simulink model "LabFabSim2022a__2_9_2023_AllAttacks_"  (R2022a)
settings: Solver=VariableStepAuto  StartTime=0.0  StopTime=5500000  RelTol=1e-3  EnableMultiTasking=on
model workspace (MAT data in the model file):
  JsonData : timetable (value not decoded)
  M : Simulink.Parameter (value not decoded)
  ROS_trigger = 0
  SL_ROS_VariableLengthArrays_MaxSizes : object (value not decoded)
undefined symbols (not defined in the file): DOS, DOSinitGen, DTP, DTPGen, DTPInitGen, EmptyLocFound, InitCobot, InitCobotReturn, InitializeSLD, InitLEGO, InitVGRproc2, m, MC, MCGen, MCInitGen, MO, MOGen, MOInitGen, n, NetScan, NetScanInitGen, Spying, SpyingInitGen, WS, WSGen, WSInitGen
libraries: sldelib x6
(part 3 of 4)

== system LabFabSim2022a__2_9_2023_AllAttacks_/VGR_Proc3 (Ramp) ==
  note: Published Return Postion
  note: DPS Detected <color> object
  note: VGR is Moving to DPS Color Sensor
  note: VGR is Picking Up Material from in-Processing Unit
  note: Calling cobot for <color> pick up
  LEGO_Cobot : Inport
  Cobot moves to pickup parts at the end of LEGO Process : EntityServer  InputPortMessageModes=m  OutputPortMessageModes=m  Capacity=1  ServiceTimeSource=Attribute  ServiceTimeAttributeName=LEGO_ServiceTime  EntryAction=|
      | sourceID(5); %lego
      | sourceAddress(4); %/lego_node
      | sourceType(1); %motion sensor
      | sourceLocation(2); %Expansion
      | destinationServiceAddress(5); %/listener(cobot)
      | destinationServiceType(5); %next task
      | destinationServiceLocation(2); %Expansion
      | accessedNodeAddress(4); 
      | accessedNodeType(1); %String
      | operation(3); %notify-callback
      | Normality(1); %normal
      | 
      | if entity.ColorID == 1
      |     value(38); %Calling cobot for RED pick up
      | else if entity.ColorID == 2
      |     value(39); %Calling cobot for BLUE pick up
      | else 
      |     value(40); %Calling cobot for WHITE pick up
      | end
  ColorSensor2 requests an open pos in HBW : EntityServer  InputPortMessageModes=m  OutputPortMessageModes=m  Capacity=1  ServiceTimeValue=5  ServiceCompleteAction=|
      | sourceID(2); %vgr
      | sourceAddress(2); %/vgr_node
      | sourceType(2); %Color sensor 
      | sourceLocation(1); %Fischertechnik
      | destinationServiceAddress(3); %/status update (main)
      | destinationServiceType(5); %next task
      | destinationServiceLocation(1); %Fischertechnik
      | accessedNodeAddress(3); 
      | accessedNodeType(1); %string
      | operation(3); %notify-callback
      | Normality(1); %normal
      | 
      | if entity.ColorID == 1
      |     value(25); %DPS Detectied RED object 
      | else if entity.ColorID == 2
      |     value(24); %DPS Detected BLUE Object 
      | else
      |     value(26); %DPS Detected WHITE object
      | end
  Empty Loc returned : EntityServer  InputPortMessageModes=m  OutputPortMessageModes=m  Capacity=1  ServiceTimeValue=0.2  EntryAction=EmptyLocFound();  ServiceCompleteAction=|
      | sourceID(3); %main
      | sourceAddress(3); %/status_update (main)
      | sourceType(4); %Order
      | sourceLocation(1); %FischerTechnik
      | destinationServiceAddress(2); %vgr_node
      | destinationServiceType(5); %Next Task
      | destinationServiceLocation(1); %Fischertechnik
      | accessedNodeAddress(2);
      | accessedNodeType(1); %string
      | operation(1); %read
      | value(43); %Published Return Postion
      | Normality(1); %normal
  Entity Gate : EntityGate  InputPortMessageModes=m,m  OutputPortMessageModes=m  OperatingMode=Release gate
  "Pump off; Cobot returns home and VGR picks up part " : EntityServer  InputPortMessageModes=m  OutputPortMessageModes=m  Capacity=1  ServiceTimeValue=3  ExitAction=|
      | sourceID(2); %vgr
      | sourceAddress(2); %/vgr_node
      | sourceType(1); %motion sensor
      | sourceLocation(1); %Fischertechnik
      | destinationServiceAddress(2); %/vgr_node
      | destinationServiceType(5); %next task
      | destinationServiceLocation(1); %Fischertechnik
      | accessedNodeAddress(3); 
      | accessedNodeType(2); %Boolean
      | operation(3); %notify-callback
      | value(22); %VGR is Picking Up Material from in-Processing Unit
      | Normality(1); %normal
  Pump on; Moves to VGR Ramp : EntityServer  InputPortMessageModes=m  OutputPortMessageModes=m  Capacity=1  ServiceTimeValue=10
  Simulink Function : Subsystem  TreatAsAtomicUnit=on
  VGR moves to color sensor 2 : EntityServer  InputPortMessageModes=m  OutputPortMessageModes=m  Capacity=1  ServiceTimeValue=11  ExitAction=|
      | sourceID(2); %vgr
      | sourceAddress(2); %/vgr_node
      | sourceType(5); %next task
      | sourceLocation(1); %Fischertechnik
      | destinationServiceAddress(2); %/vgr_node
      | destinationServiceType(5); %next task
      | destinationServiceLocation(1); %Fischertechnik
      | accessedNodeAddress(3); 
      | accessedNodeType(1); %string
      | operation(3); %notify-callback
      | value(23); %VGR is Moving to DPS Color Sensor
      | Normality(1); %normal
  Cobot_VGR : Outport
  wires:
  Cobot moves to pickup parts at the end of LEGO Process/1 -> Pump on; Moves to VGR Ramp/1
  LEGO_Cobot/1 -> Cobot moves to pickup parts at the end of LEGO Process/1
  Pump on; Moves to VGR Ramp/1 -> "Pump off; Cobot returns home and VGR picks up part "/1
  "Pump off; Cobot returns home and VGR picks up part "/1 -> VGR moves to color sensor 2/1
  ColorSensor2 requests an open pos in HBW/1 -> Empty Loc returned/1
  Empty Loc returned/1 -> Entity Gate/2
  Simulink Function/1(Out1) -> Entity Gate/1
  Entity Gate/1 -> Cobot_VGR/1
  VGR moves to color sensor 2/1 -> ColorSensor2 requests an open pos in HBW/1

== system LabFabSim2022a__2_9_2023_AllAttacks_/WrongSetup (WS) ==
  note: SourID(2), SourAdd(2), SourType(3), SourLoc(1), Dest.Serv.Add(4), Dest.Serv.Type(1), Dest.Serv.Loc(2), Acc.Node.Add(4), Acc.Node.Type(2), Op(1), Val(48)
  note: Entity Gate:
      | set to open when a positive signal value is passed into the control port. Closes when negative.
  note: Recieve signal from Chance-setting Server block for activation signal
  note: Service Time: 1700 Timestep
  note: Generates a single entity that causes Wrong Setup attack (entity generator) to generate one entity
  note: Sets WS_id up to 6 and resets to 1 for next Wrong Setup attack
  note: On Service Completion: Send a signal to data-logging SimFunctions
  note: Service Time: 600 Timestep
  Display : Display
  Entity Gate : EntityGate  InputPortMessageModes=m,m  OutputPortMessageModes=m
  Entity Generator : EntityGenerator  InputPortMessageModes=m  OutputPortMessageModes=m  GenerationMethod=Event-based  IntergenerationTimeAction=|  GenerateAction=|  AttributeName=WS_id  EntityType=Structured  EntityTypeName=WSAttack
      IntergenerationTimeAction=|
      | chanceDOS = rand(1,1);
      | if chanceDOS < 0.3
      |     dt = 1
      GenerateAction=|
      | persistent next_id_WS
      | 
      | if isempty(next_id_WS)
      |     next_id_WS = 1;
      |     %set seed for random number generation
      |     rng(12345);
      | end
      | 
      | entity.WS_id = next_id_WS
      | next_id_WS = next_id_WS + 1
      | 
      | if entity.WS_id == 1
      |     next_id_WS = 1
      settings: InputPortMap=u0
  Entity Server : EntityServer  InputPortMessageModes=m  OutputPortMessageModes=m  Capacity=1  ServiceTimeValue=1700  ServiceCompleteAction=|
      | sourceID(2); %vgr
      | sourceAddress(2); %/vgr_node
      | sourceType(3); %Reference Switch
      | sourceLocation(1); %Fischertechnik
      | destinationServiceAddress(4); %/lego_node
      | destinationServiceType(1); %Motion Sensor
      | destinationServiceLocation(2); %Expansion
      | accessedNodeAddress(4); 
      | accessedNodeType(2); %Boolean
      | operation(1); %read
      | value(44); %False
      | Normality(3); %anomalous(wrongSetUp)
  Entity Server1 : EntityServer  InputPortMessageModes=m  OutputPortMessageModes=m  Capacity=1  ServiceTimeValue=600  ServiceCompleteAction=|
      | sourceID(2); %vgr
      | sourceAddress(2); %/vgr_node
      | sourceType(3); %Reference Switch
      | sourceLocation(1); %Fischertechnik
      | destinationServiceAddress(4); %/lego_node
      | destinationServiceType(1); %Motion Sensor
      | destinationServiceLocation(2); %Expansion
      | accessedNodeAddress(4); 
      | accessedNodeType(2); %Boolean
      | operation(1); %read
      | value(44); %Flase
      | Normality(3); %anomalous(wrongSetUp)
  Entity Store : EntityStore  InputPortMessageModes=m  OutputPortMessageModes=m  Capacity=2
      settings: OutputPortMap=o4
  Entity Terminator1 : EntityTerminator  InputPortMessageModes=m  NumberEntitiesArrived=on
      settings: OutputPortMap=o0
  InitWrongSetup : Subsystem
  "Number of Entities Generated from main " : Display
  Simulink Function1 : Subsystem  TreatAsAtomicUnit=on
  Subsystem1 : Subsystem
  Wrong Setup : Subsystem  TreatAsAtomicUnit=on
  wires:
  Simulink Function1/1(Out1) -> Entity Generator/1
  Entity Terminator1/1 -> Display/1
  Entity Generator/1 -> Entity Store/1
  Entity Store/1 -> Entity Gate/2
  Entity Server/1 -> Entity Server1/1
  Wrong Setup/1(Out1) -> Entity Gate/1
  Subsystem1/1(Out1) -> Simulink Function1/1(In1)
  InitWrongSetup/1(Out1) -> "Number of Entities Generated from main "/1
  Entity Server1/1 -> Entity Terminator1/1
  Entity Gate/1 -> Entity Server/1

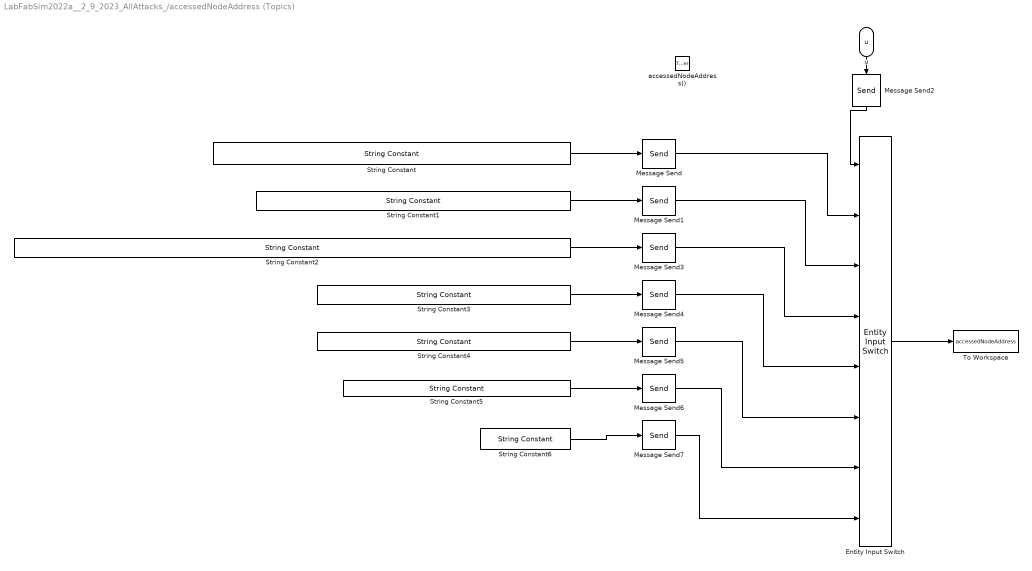
== system LabFabSim2022a__2_9_2023_AllAttacks_/accessedNodeAddress (Topics) ==
  accessedNodeAddress() : TriggerPort  TriggerType=function-call  IsSimulinkFunction=on  FunctionName=accessedNodeAddress  VariantControl=(inherit)
  Entity Input Switch : EntityInputSwitch  InputPortMessageModes=m,m,m,m,m,m,m,m  OutputPortMessageModes=m  NumberInputPorts=7  ActivePortSelection=Switch  SwitchingCriterion=From control port
      settings: InputPortMap=u0,u1,u2,u3,u4,u5,u6,u7
  Message Send{,1..7} (8 alike) : Send  OutputPortMessageModes=m
  String Constant : StringConstant  String="\"/diagnostics, /hbw_pub, /new_order, /rosout, /vgr_new_material, /what_is_empty, /what_is_occupied\""
  String Constant1 : StringConstant  String="\"/provide_empty_loc, /provide_empty_loc_back, /rosout, /what_is_empty, /what_is_occupied\""
  String Constant2 : StringConstant  String="\"/diagnostics, /new_order, /provide_empty_loc, /provide_empty_loc_back, /rosout, /sld_blue_pub, /sld_red_pub, /sld_white_pub, /vgr_drop_off, /vgr_new_material, /vgr_pub\""
  String Constant3 : StringConstant  String="\"/diagnostics, /lego_blue_pub, /lego_red_pub, /lego_white_pub, /rosout \""
  String Constant4 : StringConstant  String="\"/lego_blue_pub, /lego_red_pub, /lego_white_pub, /rosout, /vgr_drop_off \""
  String Constant5 : StringConstant  String="\"/provide_empty_loc, /rosout, /what_is_empty, /what_is_occupied\""
  String Constant6 : StringConstant  String="\"/new_order, /rosout\""
  To Workspace : ToWorkspace  VariableName=accessedNodeAddress  SaveFormat=Timeseries  SampleTime=-1
  u : ArgIn  DisableCoverage=on  ArgumentName=u
  wires:
  Entity Input Switch/1 -> To Workspace/1
  Message Send2/1 -> Entity Input Switch/1
  u/1 -> Message Send2/1
  String Constant6/1 -> Message Send7/1
  String Constant4/1 -> Message Send5/1
  String Constant/1 -> Message Send/1
  String Constant3/1 -> Message Send4/1
  String Constant2/1 -> Message Send3/1
  String Constant1/1 -> Message Send1/1
  String Constant5/1 -> Message Send6/1
  Message Send/1 -> Entity Input Switch/2
  Message Send1/1 -> Entity Input Switch/3
  Message Send3/1 -> Entity Input Switch/4
  Message Send4/1 -> Entity Input Switch/5
  Message Send5/1 -> Entity Input Switch/6
  Message Send6/1 -> Entity Input Switch/7
  Message Send7/1 -> Entity Input Switch/8

== system LabFabSim2022a__2_9_2023_AllAttacks_/accessedNodeType ==
  accessedNodeType() : TriggerPort  TriggerType=function-call  IsSimulinkFunction=on  FunctionName=accessedNodeType  VariantControl=(inherit)
  Entity Input Switch : EntityInputSwitch  InputPortMessageModes=m,m,m,m  OutputPortMessageModes=m  NumberInputPorts=3  ActivePortSelection=Switch  SwitchingCriterion=From control port
      settings: InputPortMap=u0,u1,u2,u3
  Message Send{,1..3} (4 alike) : Send  OutputPortMessageModes=m
  String Constant : StringConstant  String="\"String\""
  String Constant1 : StringConstant  String="\"Boolean\""
  String Constant2 : StringConstant  String="\"Integer\""
  To Workspace : ToWorkspace  VariableName=accessedNodeType  SaveFormat=Timeseries  SampleTime=-1
  u : ArgIn  DisableCoverage=on  ArgumentName=u
  wires:
  String Constant2/1 -> Message Send3/1
  u/1 -> Message Send2/1
  String Constant/1 -> Message Send/1
  Message Send2/1 -> Entity Input Switch/1
  String Constant1/1 -> Message Send1/1
  Entity Input Switch/1 -> To Workspace/1
  Message Send/1 -> Entity Input Switch/2
  Message Send1/1 -> Entity Input Switch/3
  Message Send3/1 -> Entity Input Switch/4

== system LabFabSim2022a__2_9_2023_AllAttacks_/destinationServiceAddress (Sub Node Name) ==
  destinationServiceAddress() : TriggerPort  TriggerType=function-call  IsSimulinkFunction=on  FunctionName=destinationServiceAddress  VariantControl=(inherit)
  Entity Input Switch : EntityInputSwitch  InputPortMessageModes=m,m,m,m,m,m  OutputPortMessageModes=m  NumberInputPorts=5  ActivePortSelection=Switch  SwitchingCriterion=From control port
      settings: InputPortMap=u0,u1,u2,u3,u4,u5
  Message Send{,1..3,5,7} (6 alike) : Send  OutputPortMessageModes=m
  String Constant : StringConstant  String="\"/hbw_node\""
  String Constant1 : StringConstant  String="\"/vgr_node\""
  String Constant2 : StringConstant  String="\"/status_update (main)\""
  String Constant4 : StringConstant  String="\"/lego_node\""
  String Constant6 : StringConstant  String="\"/listener (Cobot)\""
  To Workspace : ToWorkspace  VariableName=destinationServiceAddress  SaveFormat=Timeseries  SampleTime=-1
  u : ArgIn  DisableCoverage=on  ArgumentName=u
  wires:
  Entity Input Switch/1 -> To Workspace/1
  Message Send2/1 -> Entity Input Switch/1
  u/1 -> Message Send2/1
  String Constant4/1 -> Message Send5/1
  String Constant1/1 -> Message Send1/1
  String Constant/1 -> Message Send/1
  String Constant2/1 -> Message Send3/1
  String Constant6/1 -> Message Send7/1
  Message Send/1 -> Entity Input Switch/2
  Message Send1/1 -> Entity Input Switch/3
  Message Send3/1 -> Entity Input Switch/4
  Message Send5/1 -> Entity Input Switch/5
  Message Send7/1 -> Entity Input Switch/6

== system LabFabSim2022a__2_9_2023_AllAttacks_/destinationServiceLocation ==
  destinationServiceLocation() : TriggerPort  TriggerType=function-call  IsSimulinkFunction=on  FunctionName=destinationServiceLocation  VariantControl=(inherit)
  Entity Input Switch : EntityInputSwitch  InputPortMessageModes=m,m,m  OutputPortMessageModes=m  ActivePortSelection=Switch  SwitchingCriterion=From control port
      settings: InputPortMap=u0,u1,u2
  Message Send : Send  OutputPortMessageModes=m
  Message Send2 : Send  OutputPortMessageModes=m
  Message Send3 : Send  OutputPortMessageModes=m
  String Constant : StringConstant  String="\"FischerTechnik\""
  String Constant2 : StringConstant  String="\"Expansion\""
  To Workspace : ToWorkspace  VariableName=destinationServiceLocation  SaveFormat=Timeseries  SampleTime=-1
  u : ArgIn  DisableCoverage=on  ArgumentName=u
  wires:
  u/1 -> Message Send2/1
  Message Send2/1 -> Entity Input Switch/1
  Entity Input Switch/1 -> To Workspace/1
  String Constant/1 -> Message Send/1
  String Constant2/1 -> Message Send3/1
  Message Send/1 -> Entity Input Switch/2
  Message Send3/1 -> Entity Input Switch/3

== system LabFabSim2022a__2_9_2023_AllAttacks_/destinationServiceType ==
  destinationServiceType() : TriggerPort  TriggerType=function-call  IsSimulinkFunction=on  FunctionName=destinationServiceType  VariantControl=(inherit)
  Entity Input Switch : EntityInputSwitch  InputPortMessageModes=m,m,m,m,m,m  OutputPortMessageModes=m  NumberInputPorts=5  ActivePortSelection=Switch  SwitchingCriterion=From control port
      settings: InputPortMap=u0,u1,u2,u3,u4,u5
  Message Send{1..3,8..10} (6 alike) : Send  OutputPortMessageModes=m
  String Constant1 : StringConstant  String="\"Order\""
  String Constant2 : StringConstant  String="\"Next Task\""
  String Constant7 : StringConstant  String="\"Motion Sensor\""
  String Constant8 : StringConstant  String="\"Color Sensor\""
  String Constant9 : StringConstant  String="\"Reference Switch\""
  To Workspace : ToWorkspace  VariableName=destinationServiceType  SaveFormat=Timeseries  SampleTime=-1
  u : ArgIn  DisableCoverage=on  ArgumentName=u
  wires:
  u/1 -> Message Send2/1
  Message Send2/1 -> Entity Input Switch/1
  Entity Input Switch/1 -> To Workspace/1
  String Constant7/1 -> Message Send8/1
  String Constant9/1 -> Message Send10/1
  String Constant8/1 -> Message Send9/1
  String Constant1/1 -> Message Send1/1
  String Constant2/1 -> Message Send3/1
  Message Send8/1 -> Entity Input Switch/2
  Message Send9/1 -> Entity Input Switch/3
  Message Send10/1 -> Entity Input Switch/4
  Message Send1/1 -> Entity Input Switch/5
  Message Send3/1 -> Entity Input Switch/6

== system LabFabSim2022a__2_9_2023_AllAttacks_/operation ==
  operation() : TriggerPort  TriggerType=function-call  IsSimulinkFunction=on  FunctionName=operation  VariantControl=(inherit)
  Entity Input Switch : EntityInputSwitch  InputPortMessageModes=m,m,m,m,m,m  OutputPortMessageModes=m  NumberInputPorts=5  ActivePortSelection=Switch  SwitchingCriterion=From control port
      settings: InputPortMap=u0,u1,u2,u3,u4,u5
  Message Send{1..6} (6 alike) : Send  OutputPortMessageModes=m
  String Constant1 : StringConstant  String="\"register/unregister service\""
  String Constant2 : StringConstant  String="\"read\""
  String Constant3 : StringConstant  String="\"subscribe/unsubscribe\""
  String Constant4 : StringConstant  String="\"notify-callback\""
  String Constant5 : StringConstant  String="\"write\""
  To Workspace : ToWorkspace  VariableName=operation  SaveFormat=Timeseries  SampleTime=-1
  u : ArgIn  DisableCoverage=on  ArgumentName=u
  wires:
  String Constant4/1 -> Message Send5/1
  String Constant3/1 -> Message Send4/1
  String Constant2/1 -> Message Send3/1
  u/1 -> Message Send2/1
  Message Send2/1 -> Entity Input Switch/1
  Entity Input Switch/1 -> To Workspace/1
  String Constant1/1 -> Message Send1/1
  Message Send3/1 -> Entity Input Switch/2
  Message Send4/1 -> Entity Input Switch/3
  Message Send5/1 -> Entity Input Switch/4
  Message Send1/1 -> Entity Input Switch/5
  Message Send6/1 -> Entity Input Switch/6
  String Constant5/1 -> Message Send6/1

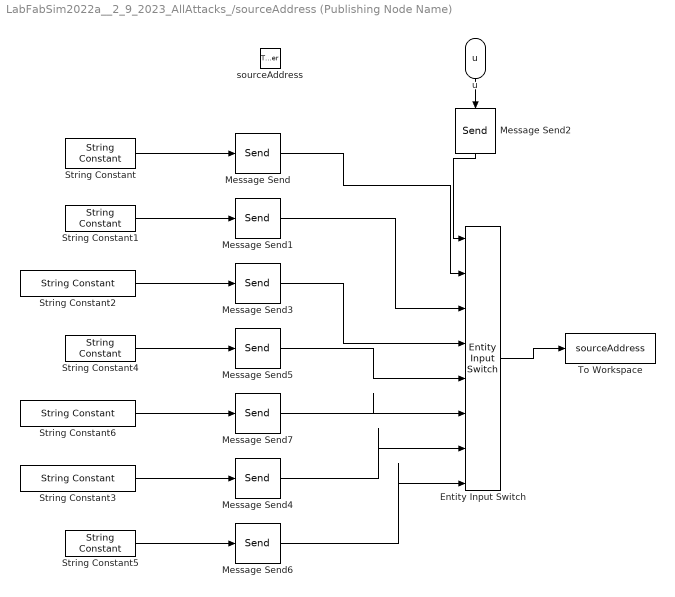
== system LabFabSim2022a__2_9_2023_AllAttacks_/sourceAddress (Publishing Node Name) ==
  sourceAddress : TriggerPort  TriggerType=function-call  IsSimulinkFunction=on  FunctionName=sourceAddress  VariantControl=(inherit)
  Entity Input Switch : EntityInputSwitch  InputPortMessageModes=m,m,m,m,m,m,m,m  OutputPortMessageModes=m  NumberInputPorts=7  ActivePortSelection=Switch  SwitchingCriterion=From control port
      settings: InputPortMap=u0,u1,u2,u3,u4,u5,u6,u7
  Message Send{,1..7} (8 alike) : Send  OutputPortMessageModes=m
  String Constant : StringConstant  String="\"/hbw_node\""
  String Constant1 : StringConstant  String="\"/vgr_node\""
  String Constant2 : StringConstant  String="\"/status_update (main)\""
  String Constant3 : StringConstant  String="\"/Order\""
  String Constant4 : StringConstant  String="\"/lego_node\""
  String Constant5 : StringConstant  String="\"/sld_node\""
  String Constant6 : StringConstant  String="\"/listener (Cobot)\""
  To Workspace : ToWorkspace  VariableName=sourceAddress  SaveFormat=Timeseries  SampleTime=-1
  u : ArgIn  DisableCoverage=on  ArgumentName=u
  wires:
  Entity Input Switch/1 -> To Workspace/1
  Message Send2/1 -> Entity Input Switch/1
  u/1 -> Message Send2/1
  String Constant1/1 -> Message Send1/1
  String Constant2/1 -> Message Send3/1
  String Constant/1 -> Message Send/1
  String Constant4/1 -> Message Send5/1
  String Constant6/1 -> Message Send7/1
  String Constant3/1 -> Message Send4/1
  Message Send/1 -> Entity Input Switch/2
  Message Send1/1 -> Entity Input Switch/3
  Message Send3/1 -> Entity Input Switch/4
  Message Send5/1 -> Entity Input Switch/5
  Message Send7/1 -> Entity Input Switch/6
  Message Send4/1 -> Entity Input Switch/7
  String Constant5/1 -> Message Send6/1
  Message Send6/1 -> Entity Input Switch/8

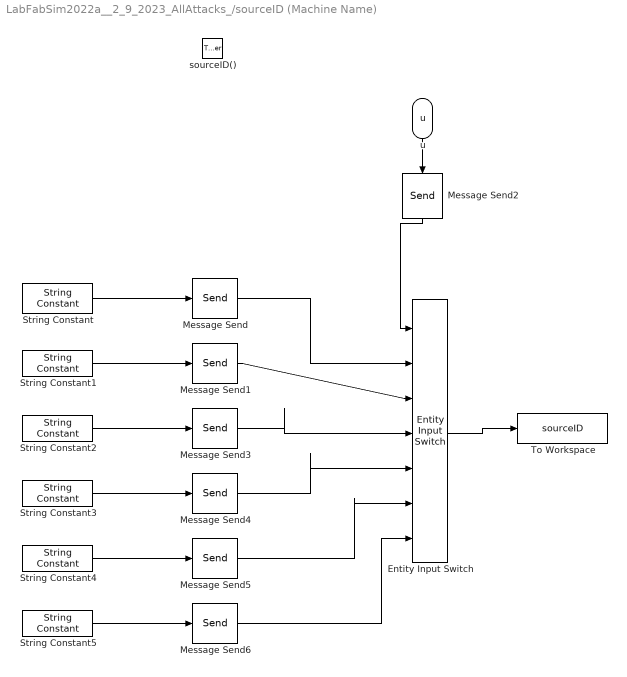
== system LabFabSim2022a__2_9_2023_AllAttacks_/sourceID (Machine Name) ==
  sourceID() : TriggerPort  TriggerType=function-call  IsSimulinkFunction=on  FunctionName=sourceID  VariantControl=(inherit)
  Entity Input Switch : EntityInputSwitch  InputPortMessageModes=m,m,m,m,m,m,m  OutputPortMessageModes=m  NumberInputPorts=6  ActivePortSelection=Switch  SwitchingCriterion=From control port
      settings: InputPortMap=u0,u1,u2,u3,u4,u5,u6
  Message Send{,1..6} (7 alike) : Send  OutputPortMessageModes=m
  String Constant : StringConstant  String="\"hbw\""
  String Constant1 : StringConstant  String="\"vgr\""
  String Constant2 : StringConstant  String="\"main\""
  String Constant3 : StringConstant  String="\"sld\""
  String Constant4 : StringConstant  String="\"lego\""
  String Constant5 : StringConstant  String="\"cobot\""
  To Workspace : ToWorkspace  VariableName=sourceID  SaveFormat=Timeseries  SampleTime=-1
  u : ArgIn  DisableCoverage=on  ArgumentName=u
  wires:
  String Constant3/1 -> Message Send4/1
  String Constant2/1 -> Message Send3/1
  u/1 -> Message Send2/1
  String Constant/1 -> Message Send/1
  Message Send2/1 -> Entity Input Switch/1
  String Constant1/1 -> Message Send1/1
  Entity Input Switch/1 -> To Workspace/1
  String Constant4/1 -> Message Send5/1
  String Constant5/1 -> Message Send6/1
  Message Send/1 -> Entity Input Switch/2
  Message Send1/1 -> Entity Input Switch/3
  Message Send3/1 -> Entity Input Switch/4
  Message Send4/1 -> Entity Input Switch/5
  Message Send5/1 -> Entity Input Switch/6
  Message Send6/1 -> Entity Input Switch/7

== system LabFabSim2022a__2_9_2023_AllAttacks_/sourceLocation ==
  sourceLocation() : TriggerPort  TriggerType=function-call  IsSimulinkFunction=on  FunctionName=sourceLocation  VariantControl=(inherit)
  Entity Input Switch : EntityInputSwitch  InputPortMessageModes=m,m,m,m  OutputPortMessageModes=m  NumberInputPorts=3  ActivePortSelection=Switch  SwitchingCriterion=From control port
      settings: InputPortMap=u0,u1,u2,u3
  Message Send{,1..3} (4 alike) : Send  OutputPortMessageModes=m
  String Constant : StringConstant  String="\"FischerTechnik\""
  String Constant1 : StringConstant  String="\"SCADA system\""
  String Constant2 : StringConstant  String="\"Expansion\""
  To Workspace : ToWorkspace  VariableName=sourceLocation  SaveFormat=Timeseries  SampleTime=-1
  u : ArgIn  DisableCoverage=on  ArgumentName=u
  wires:
  String Constant2/1 -> Message Send3/1
  u/1 -> Message Send2/1
  String Constant/1 -> Message Send/1
  Message Send2/1 -> Entity Input Switch/1
  Entity Input Switch/1 -> To Workspace/1
  String Constant1/1 -> Message Send1/1
  Message Send1/1 -> Entity Input Switch/4
  Message Send3/1 -> Entity Input Switch/3
  Message Send/1 -> Entity Input Switch/2

== system LabFabSim2022a__2_9_2023_AllAttacks_/sourceType ==
  sourceType() : TriggerPort  TriggerType=function-call  IsSimulinkFunction=on  FunctionName=sourceType  VariantControl=(inherit)
  Entity Input Switch : EntityInputSwitch  InputPortMessageModes=m,m,m,m,m,m  OutputPortMessageModes=m  NumberInputPorts=5  ActivePortSelection=Switch  SwitchingCriterion=From control port
      settings: InputPortMap=u0,u1,u2,u3,u4,u5
  Message Send{,1..5} (6 alike) : Send  OutputPortMessageModes=m
  String Constant : StringConstant  String="\"Motion Sensor\""
  String Constant1 : StringConstant  String="\"Color Sensor\""
  String Constant2 : StringConstant  String="\"Reference Switch\""
  String Constant3 : StringConstant  String="\"Order\""
  String Constant4 : StringConstant  String="\"Next Task\""
  To Workspace : ToWorkspace  VariableName=sourceType  SaveFormat=Timeseries  SampleTime=-1
  u : ArgIn  DisableCoverage=on  ArgumentName=u
  wires:
  Entity Input Switch/1 -> To Workspace/1
  String Constant1/1 -> Message Send1/1
  Message Send2/1 -> Entity Input Switch/1
  String Constant/1 -> Message Send/1
  u/1 -> Message Send2/1
  String Constant2/1 -> Message Send3/1
  String Constant3/1 -> Message Send5/1
  String Constant4/1 -> Message Send4/1
  Message Send/1 -> Entity Input Switch/2
  Message Send1/1 -> Entity Input Switch/3
  Message Send3/1 -> Entity Input Switch/4
  Message Send5/1 -> Entity Input Switch/5
  Message Send4/1 -> Entity Input Switch/6

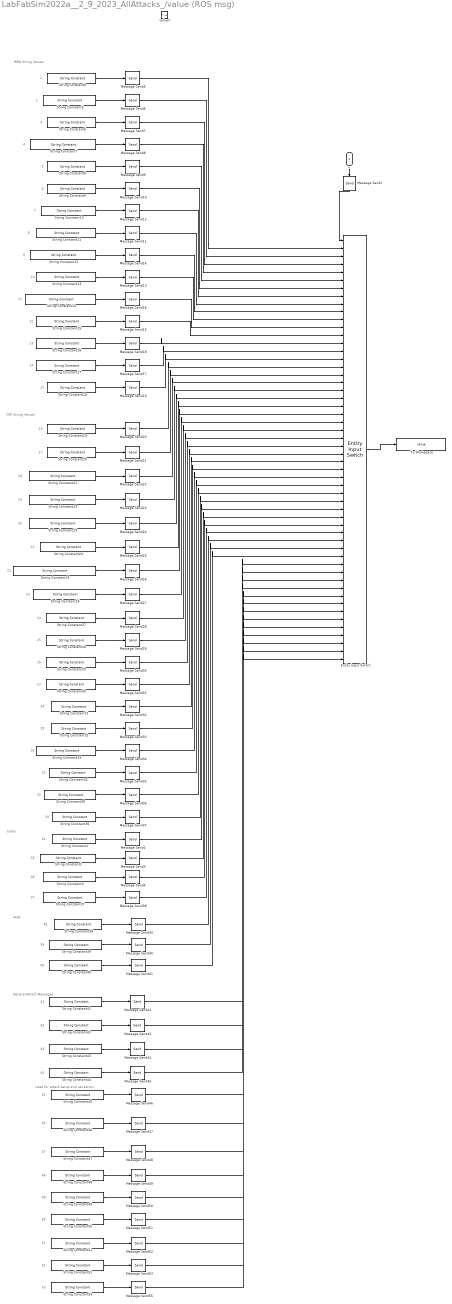
== system LabFabSim2022a__2_9_2023_AllAttacks_/value (ROS msg) ==
  note: General/Attack Messages
  note: Used for attack setup and validation
  note: Lego
  note: Cobot
  note: 1
  note: VGR String Values
  note: HBW String Values
  note: 2
  note: 3
  note: 4
  note: 5
  note: 6
  note: 7
  note: 8
  note: 9
  note: 10
  note: 11
  note: 12
  note: 13
  note: 14
  note: 15
  note: 16
  note: 17
  note: 18
  note: 19
  note: 20
  note: 21
  note: 22
  note: 23
  note: 24
  note: 25
  note: 26
  note: 27
  note: 28
  note: 29
  note: 30
  note: 31
  note: 32
  note: 33
  note: 34
  note: 35
  note: 36
  note: 37
  note: 38
  note: 39
  note: 40
  note: 41
  note: 42
  note: 43
  note: 44
  note: 45
  note: 46
  note: 47
  note: 48
  note: 49
  note: 50
  note: 51
  note: 52
  note: 53
  value() : TriggerPort  TriggerType=function-call  IsSimulinkFunction=on  FunctionName=value  VariantControl=(inherit)
  Entity Input Switch : EntityInputSwitch  InputPortMessageModes=m,m,m,m,m,m,m,m,m,m,m,m,m,m,m,m,m,m,m,m,m,m,m,m,m,m,m,m,m,m,m,m,m,m,m,m,m,m,m,m,m,m,m,m,m,m,m,m,m,m,m,m,m,m  OutputPortMessageModes=m  NumberInputPorts=53  ActivePortSelection=Switch  SwitchingCriterion=From control port
      settings: InputPortMap=u0,u1,u2,u3,u4,u5,u6,u7,u8,u9,u10,u11,u12,u13,u14,u15,u16,u17,u18,u19,u20,u21,u22,u23,u24,u25,u26,u27,u28,u29,u30,u31,u32,u33,u34,u35,u36,u37,u38,u39,u40,u41,u42,u43,u44,u45,u46,u47,u48,u49,u50,u51,u52,u53
  Message Send{1..53,55} (54 alike) : Send  OutputPortMessageModes=m
  String Constant1 : StringConstant  String="\"Order is ready for picking\""
  String Constant10 : StringConstant  String="\"HBW Material is Picked by VGR\""
  String Constant11 : StringConstant  String="\"HBW Material is Dropped by VGR\""
  String Constant12 : StringConstant  String="\"Empty Box is Ready for HBW Pick Up\""
  String Constant13 : StringConstant  String="\"Material is Ready for HBW Pick Up\""
  String Constant14 : StringConstant  String="\"HBW Picked up the Empty Box from the Belt\""
  String Constant15 : StringConstant  String="\"HBW Picked up Material from the Belt\""
  String Constant16 : StringConstant  String="\"HBW Empty Box is Back on the Shelf\""
  String Constant17 : StringConstant  String="\"HBW Placed Material on the Shelf\""
  String Constant18 : StringConstant  String="\"HBW Robot is Set to Home\""
  String Constant19 : StringConstant  String="\"VGR is Set to Home\""
  String Constant2 : StringConstant  String="\"Red order is ready for pick up\""
  String Constant20 : StringConstant  String="\"VGR Dropped Material at DPS\""
  String Constant21 : StringConstant  String="\"VGR Received an Order at the BLUE Topic\""
  String Constant22 : StringConstant  String="\"VGR Received an Order at the RED Topic\""
  String Constant23 : StringConstant  String="\"VGR Received an Order at the WHITE Topic\""
  String Constant24 : StringConstant  String="\"VGR Dropped Material at HBW\""
  String Constant25 : StringConstant  String="\"VGR is Picking Up Material from in-Processing Unit\""
  String Constant26 : StringConstant  String="\"VGR is Moving to DPS Color Sensor\""
  String Constant27 : StringConstant  String="\"DPS Detected Blue Object\""
  String Constant28 : StringConstant  String="\"DPS Detected Red Object\""
  String Constant29 : StringConstant  String="\"DPS Detected White Object\""
  String Constant3 : StringConstant  String="\"Blue order is ready for pick up\""
  String Constant30 : StringConstant  String="\"vgr asks for free location\""
  String Constant31 : StringConstant  String="\"VGR got something\""
  String Constant32 : StringConstant  String="\"VGR is Moving to HBW\""
  String Constant33 : StringConstant  String="\"VGR Picked Up Material from HBW\""
  String Constant34 : StringConstant  String="\"VGR is Moving to MPS\""
  String Constant35 : StringConstant  String="\"VGR Dropped Material at MPS\""
  String Constant36 : StringConstant  String="\"Calling Cobot for Picking\""
  String Constant37 : StringConstant  String="\"White order is ready for pick up\""
  String Constant38 : StringConstant  String="\"Calling Cobot for red Pick up\""
  String Constant39 : StringConstant  String="\"Calling Cobot for blue Pick up\""
  String Constant4 : StringConstant  String="\"HBW Recieved an Order\""
  String Constant40 : StringConstant  String="\"Calling Cobot for white Pick up\""
  String Constant41 : StringConstant  String="\"Published Order\""
  String Constant42 : StringConstant  String="\"Status Updated Successfully\""
  String Constant43 : StringConstant  String="\"Published Return Position\""
  String Constant44 : StringConstant  String="\"0\""
  String Constant45 : StringConstant  String="\"Spy\""
  String Constant46 : StringConstant  String="\"DTP\""
  String Constant47 : StringConstant  String="\"MO\""
  String Constant48 : StringConstant  String="\"WS\""
  String Constant49 : StringConstant  String="\"MC\""
  String Constant5 : StringConstant  String="\"HBW is Preparing an Empty Box\""
  String Constant50 : StringConstant  String="\"1\""
  String Constant51 : StringConstant  String="\"Cobot Idle\""
  String Constant52 : StringConstant  String="\"N/A\""
  String Constant53 : StringConstant  String="\" \""
  String Constant6 : StringConstant  String="\"HBW Picked Up Material\""
  String Constant7 : StringConstant  String="\"HBW Picked Empty Box from The Shelf\""
  String Constant8 : StringConstant  String="\"HBW Placed Material on Belt\""
  String Constant9 : StringConstant  String="\"HBW Placed Box on the Belt\""
  To Workspace : ToWorkspace  VariableName=value  SaveFormat=Timeseries  SampleTime=-1
  u : ArgIn  DisableCoverage=on  ArgumentName=u
  wires:
  u/1 -> Message Send2/1
  Message Send2/1 -> Entity Input Switch/1
  Entity Input Switch/1 -> To Workspace/1
  String Constant4/1 -> Message Send5/1
  String Constant5/1 -> Message Send6/1
  String Constant6/1 -> Message Send7/1
  String Constant7/1 -> Message Send8/1
  String Constant8/1 -> Message Send9/1
  String Constant9/1 -> Message Send10/1
  String Constant11/1 -> Message Send11/1
  String Constant10/1 -> Message Send12/1
  String Constant12/1 -> Message Send14/1
  String Constant13/1 -> Message Send13/1
  String Constant15/1 -> Message Send15/1
  String Constant14/1 -> Message Send16/1
  String Constant16/1 -> Message Send18/1
  String Constant17/1 -> Message Send17/1
  String Constant18/1 -> Message Send19/1
  String Constant19/1 -> Message Send20/1
  String Constant20/1 -> Message Send21/1
  String Constant21/1 -> Message Send22/1
  String Constant22/1 -> Message Send23/1
  String Constant23/1 -> Message Send24/1
  String Constant24/1 -> Message Send25/1
  String Constant25/1 -> Message Send26/1
  String Constant26/1 -> Message Send27/1
  String Constant27/1 -> Message Send28/1
  String Constant28/1 -> Message Send29/1
  String Constant29/1 -> Message Send30/1
  String Constant30/1 -> Message Send31/1
  String Constant31/1 -> Message Send32/1
  String Constant32/1 -> Message Send33/1
  String Constant33/1 -> Message Send34/1
  String Constant34/1 -> Message Send35/1
  String Constant35/1 -> Message Send36/1
  String Constant36/1 -> Message Send37/1
  String Constant1/1 -> Message Send1/1
  String Constant2/1 -> Message Send3/1
  String Constant3/1 -> Message Send4/1
  String Constant37/1 -> Message Send38/1
  String Constant38/1 -> Message Send39/1
  String Constant39/1 -> Message Send40/1
  String Constant40/1 -> Message Send41/1
  String Constant41/1 -> Message Send42/1
  String Constant42/1 -> Message Send43/1
  String Constant43/1 -> Message Send44/1
  Message Send5/1 -> Entity Input Switch/2
  Message Send6/1 -> Entity Input Switch/3
  Message Send7/1 -> Entity Input Switch/4
  Message Send8/1 -> Entity Input Switch/5
  Message Send9/1 -> Entity Input Switch/6
  Message Send10/1 -> Entity Input Switch/7
  Message Send12/1 -> Entity Input Switch/8
  Message Send11/1 -> Entity Input Switch/9
  Message Send14/1 -> Entity Input Switch/10
  Message Send13/1 -> Entity Input Switch/11
  Message Send16/1 -> Entity Input Switch/12
  Message Send15/1 -> Entity Input Switch/13
  Message Send18/1 -> Entity Input Switch/14
  Message Send17/1 -> Entity Input Switch/15
  Message Send19/1 -> Entity Input Switch/16
  Message Send20/1 -> Entity Input Switch/17
  Message Send21/1 -> Entity Input Switch/18
  Message Send22/1 -> Entity Input Switch/19
  Message Send23/1 -> Entity Input Switch/20
  Message Send24/1 -> Entity Input Switch/21
  Message Send25/1 -> Entity Input Switch/22
  Message Send26/1 -> Entity Input Switch/23
  Message Send27/1 -> Entity Input Switch/24
  Message Send28/1 -> Entity Input Switch/25
  Message Send29/1 -> Entity Input Switch/26
  Message Send30/1 -> Entity Input Switch/27
  Message Send31/1 -> Entity Input Switch/28
  Message Send32/1 -> Entity Input Switch/29
  Message Send33/1 -> Entity Input Switch/30
  Message Send34/1 -> Entity Input Switch/31
  Message Send35/1 -> Entity Input Switch/32
  Message Send36/1 -> Entity Input Switch/33
  Message Send37/1 -> Entity Input Switch/34
  Message Send1/1 -> Entity Input Switch/35
  Message Send3/1 -> Entity Input Switch/36
  Message Send4/1 -> Entity Input Switch/37
  Message Send38/1 -> Entity Input Switch/38
  Message Send39/1 -> Entity Input Switch/39
  Message Send40/1 -> Entity Input Switch/40
  Message Send41/1 -> Entity Input Switch/41
  Message Send42/1 -> Entity Input Switch/42
  Message Send43/1 -> Entity Input Switch/43
  Message Send44/1 -> Entity Input Switch/44
  Message Send45/1 -> Entity Input Switch/45
  String Constant44/1 -> Message Send45/1
  String Constant45/1 -> Message Send46/1
  Message Send46/1 -> Entity Input Switch/46
  String Constant46/1 -> Message Send47/1
  Message Send47/1 -> Entity Input Switch/47
  Message Send48/1 -> Entity Input Switch/48
  String Constant47/1 -> Message Send48/1
  String Constant48/1 -> Message Send49/1
  Message Send49/1 -> Entity Input Switch/49
  Message Send50/1 -> Entity Input Switch/50
  String Constant49/1 -> Message Send50/1
  String Constant50/1 -> Message Send51/1
  Message Send51/1 -> Entity Input Switch/51
  Message Send52/1 -> Entity Input Switch/52
  String Constant51/1 -> Message Send52/1
  String Constant52/1 -> Message Send53/1
  Message Send53/1 -> Entity Input Switch/53
  Message Send55/1 -> Entity Input Switch/54
  String Constant53/1 -> Message Send55/1

== system LabFabSim2022a__2_9_2023_AllAttacks_/Cobot_LEGO/Simulink Function ==
  InitLEGO() : TriggerPort  TriggerType=function-call  IsSimulinkFunction=on  FunctionName=InitLEGO  VariantControl=(inherit)
  Constant : Constant
  Message Send : Send  OutputPortMessageModes=m
  Out1 : Outport
  wires:
  Constant/1 -> Message Send/1
  Message Send/1 -> Out1/1

== system LabFabSim2022a__2_9_2023_AllAttacks_/DOS/DOS ==
  DOS : TriggerPort  TriggerType=function-call  IsSimulinkFunction=on  FunctionName=DOS  VariantControl=(inherit)
  Message Send : Send  OutputPortMessageModes=m
  u : ArgIn  DisableCoverage=on  ArgumentName=u
  Out1 : Outport
  wires:
  u/1 -> Message Send/1
  Message Send/1 -> Out1/1

== system LabFabSim2022a__2_9_2023_AllAttacks_/DOS/InitDOS ==
  note: On Entry: Generate 400 DOS attack entities
  Entity Generator1 : EntityGenerator  InputPortMessageModes=m  OutputPortMessageModes=m  GenerationMethod=Event-based  Period=inf  AttributeName=data  EntityType=Structured  EntityTypeName=InitDOS
      settings: InputPortMap=u0
  Entity Terminator2 : EntityTerminator  InputPortMessageModes=m  EntryAction=|  NumberEntitiesArrived=on
      | for i = 1:400
      |     DOSgen();
      | end
      settings: OutputPortMap=o0
  Simulink Function2 : Subsystem  TreatAsAtomicUnit=on
  Subsystem2 : Subsystem
  Out1 : Outport
  wires:
  Subsystem2/1(Out1) -> Simulink Function2/1(In1)
  Simulink Function2/1(Out1) -> Entity Generator1/1
  Entity Terminator2/1 -> Out1/1
  Entity Generator1/1 -> Entity Terminator2/1

== system LabFabSim2022a__2_9_2023_AllAttacks_/DOS/Simulink Function1 ==
  In1 : Inport
  DOSgen : TriggerPort  TriggerType=function-call  IsSimulinkFunction=on  FunctionName=DOSgen  VariantControl=(inherit)
  Message Send : Send  OutputPortMessageModes=m
  Out1 : Outport
  wires:
  Message Send/1 -> Out1/1
  In1/1 -> Message Send/1

== system LabFabSim2022a__2_9_2023_AllAttacks_/DOS/Subsystem1 ==
  Constant : Constant
  Out1 : Outport
  wires:
  Constant/1 -> Out1/1

== system LabFabSim2022a__2_9_2023_AllAttacks_/DataTypesProbing (DTP)/InitDataTypesProbing ==
  note: On Entry: Generate 1 DataTypesProbing attack entities
  Entity Generator1 : EntityGenerator  InputPortMessageModes=m  OutputPortMessageModes=m  GenerationMethod=Event-based  Period=inf  AttributeName=data  EntityType=Structured  EntityTypeName=InitDTP
      settings: InputPortMap=u0
  Entity Terminator2 : EntityTerminator  InputPortMessageModes=m  EntryAction=DTPGen();  NumberEntitiesArrived=on
      settings: OutputPortMap=o0
  Simulink Function2 : Subsystem  TreatAsAtomicUnit=on
  Subsystem2 : Subsystem
  Out1 : Outport
  wires:
  Subsystem2/1(Out1) -> Simulink Function2/1(In1)
  Simulink Function2/1(Out1) -> Entity Generator1/1
  Entity Terminator2/1 -> Out1/1
  Entity Generator1/1 -> Entity Terminator2/1

== system LabFabSim2022a__2_9_2023_AllAttacks_/DataTypesProbing (DTP)/Simulink Function1 ==
  In1 : Inport
  DTPGen : TriggerPort  TriggerType=function-call  IsSimulinkFunction=on  FunctionName=DTPGen  VariantControl=(inherit)
  Message Send : Send  OutputPortMessageModes=m
  Out1 : Outport
  wires:
  Message Send/1 -> Out1/1
  In1/1 -> Message Send/1

== system LabFabSim2022a__2_9_2023_AllAttacks_/DataTypesProbing (DTP)/Spying ==
  DTP : TriggerPort  TriggerType=function-call  IsSimulinkFunction=on  FunctionName=DTP  VariantControl=(inherit)
  Message Send : Send  OutputPortMessageModes=m
  u : ArgIn  DisableCoverage=on  ArgumentName=u
  Out1 : Outport
  wires:
  u/1 -> Message Send/1
  Message Send/1 -> Out1/1

== system LabFabSim2022a__2_9_2023_AllAttacks_/DataTypesProbing (DTP)/Subsystem1 ==
  Constant : Constant
  Out1 : Outport
  wires:
  Constant/1 -> Out1/1

== system LabFabSim2022a__2_9_2023_AllAttacks_/HBW_Start (DOS)/Simulink Function ==
  VGR_PickupPart() : TriggerPort  TriggerType=function-call  IsSimulinkFunction=on  FunctionName=VGR_PickupPart  VariantControl=(inherit)
  Constant : Constant
  Message Send : Send  OutputPortMessageModes=m
  Out1 : Outport
  wires:
  Constant/1 -> Message Send/1
  Message Send/1 -> Out1/1

== system LabFabSim2022a__2_9_2023_AllAttacks_/HBW_Start (DOS)/Simulink Function2 ==
  DOS_Router : TriggerPort  TriggerType=function-call  IsSimulinkFunction=on  FunctionName=DOS_Router  VariantControl=(inherit)
  Constant : Constant  Value=2
  Constant1 : Constant
  Switch : Switch  Threshold=2  ZeroCross=off  SaturateOnIntegerOverflow=off  InputSameDT=off
  u : ArgIn  DisableCoverage=on  ArgumentName=u
  Out1 : Outport
  wires:
  u/1 -> Switch/2
  Switch/1 -> Out1/1
  Constant1/1 -> Switch/1
  Constant/1 -> Switch/3

== system LabFabSim2022a__2_9_2023_AllAttacks_/LEGO_Cobot (DTP)/Simulink Function ==
  InitCobotReturn() : TriggerPort  TriggerType=function-call  IsSimulinkFunction=on  FunctionName=InitCobotReturn  VariantControl=(inherit)
  Constant : Constant
  Message Send : Send  OutputPortMessageModes=m
  Out1 : Outport
  wires:
  Constant/1 -> Message Send/1
  Message Send/1 -> Out1/1

== system LabFabSim2022a__2_9_2023_AllAttacks_/LEGO_Cobot (DTP)/Simulink Function2 ==
  DTP_Router : TriggerPort  TriggerType=function-call  IsSimulinkFunction=on  FunctionName=DTP_Router  VariantControl=(inherit)
  Constant : Constant  Value=2
  Constant1 : Constant
  Switch : Switch  Threshold=2  ZeroCross=off  SaturateOnIntegerOverflow=off  InputSameDT=off
  u : ArgIn  DisableCoverage=on  ArgumentName=u
  Out1 : Outport
  wires:
  u/1 -> Switch/2
  Switch/1 -> Out1/1
  Constant1/1 -> Switch/1
  Constant/1 -> Switch/3

== system LabFabSim2022a__2_9_2023_AllAttacks_/MPS/Simulink Function ==
  InitializeSLD() : TriggerPort  TriggerType=function-call  IsSimulinkFunction=on  FunctionName=InitializeSLD  VariantControl=(inherit)
  Constant : Constant
  Message Send : Send  OutputPortMessageModes=m
  Out1 : Outport
  wires:
  Message Send/1 -> Out1/1
  Constant/1 -> Message Send/1

== system LabFabSim2022a__2_9_2023_AllAttacks_/MaliciousControl (MC)/InitMaliciousControl ==
  note: On Entry: Generate 1 Malicious Control attack entities
  Entity Generator1 : EntityGenerator  InputPortMessageModes=m  OutputPortMessageModes=m  GenerationMethod=Event-based  Period=inf  AttributeName=data  EntityType=Structured  EntityTypeName=InitMC
      settings: InputPortMap=u0
  Entity Terminator2 : EntityTerminator  InputPortMessageModes=m  EntryAction=MCGen();  NumberEntitiesArrived=on
      settings: OutputPortMap=o0
  Simulink Function2 : Subsystem  TreatAsAtomicUnit=on
  Subsystem2 : Subsystem
  Out1 : Outport
  wires:
  Subsystem2/1(Out1) -> Simulink Function2/1(In1)
  Simulink Function2/1(Out1) -> Entity Generator1/1
  Entity Terminator2/1 -> Out1/1
  Entity Generator1/1 -> Entity Terminator2/1

== system LabFabSim2022a__2_9_2023_AllAttacks_/MaliciousControl (MC)/Malicious Control ==
  MC : TriggerPort  TriggerType=function-call  IsSimulinkFunction=on  FunctionName=MC  VariantControl=(inherit)
  Message Send : Send  OutputPortMessageModes=m
  u : ArgIn  DisableCoverage=on  ArgumentName=u
  Out1 : Outport
  wires:
  u/1 -> Message Send/1
  Message Send/1 -> Out1/1

== system LabFabSim2022a__2_9_2023_AllAttacks_/MaliciousControl (MC)/Simulink Function1 ==
  In1 : Inport
  MCGen : TriggerPort  TriggerType=function-call  IsSimulinkFunction=on  FunctionName=MCGen  VariantControl=(inherit)
  Message Send : Send  OutputPortMessageModes=m
  Out1 : Outport
  wires:
  Message Send/1 -> Out1/1
  In1/1 -> Message Send/1

== system LabFabSim2022a__2_9_2023_AllAttacks_/MaliciousControl (MC)/Subsystem1 ==
  Constant : Constant
  Out1 : Outport
  wires:
  Constant/1 -> Out1/1

== system LabFabSim2022a__2_9_2023_AllAttacks_/MaliciousOperation (MO)/InitMaliciousOperation ==
  note: On Entry: Generate 1 Malicious Operation attack entities
  Entity Generator1 : EntityGenerator  InputPortMessageModes=m  OutputPortMessageModes=m  GenerationMethod=Event-based  Period=inf  AttributeName=data  EntityType=Structured  EntityTypeName=InitMO
      settings: InputPortMap=u0
  Entity Terminator2 : EntityTerminator  InputPortMessageModes=m  EntryAction=MOGen();  NumberEntitiesArrived=on
      settings: OutputPortMap=o0
  Simulink Function2 : Subsystem  TreatAsAtomicUnit=on
  Subsystem2 : Subsystem
  Out1 : Outport
  wires:
  Subsystem2/1(Out1) -> Simulink Function2/1(In1)
  Simulink Function2/1(Out1) -> Entity Generator1/1
  Entity Terminator2/1 -> Out1/1
  Entity Generator1/1 -> Entity Terminator2/1

== system LabFabSim2022a__2_9_2023_AllAttacks_/MaliciousOperation (MO)/Malicious Operation ==
  MO : TriggerPort  TriggerType=function-call  IsSimulinkFunction=on  FunctionName=MO  VariantControl=(inherit)
  Message Send : Send  OutputPortMessageModes=m
  u : ArgIn  DisableCoverage=on  ArgumentName=u
  Out1 : Outport
  wires:
  u/1 -> Message Send/1
  Message Send/1 -> Out1/1

== system LabFabSim2022a__2_9_2023_AllAttacks_/MaliciousOperation (MO)/Simulink Function1 ==
  In1 : Inport
  MOGen : TriggerPort  TriggerType=function-call  IsSimulinkFunction=on  FunctionName=MOGen  VariantControl=(inherit)
  Message Send : Send  OutputPortMessageModes=m
  Out1 : Outport
  wires:
  Message Send/1 -> Out1/1
  In1/1 -> Message Send/1

== system LabFabSim2022a__2_9_2023_AllAttacks_/MaliciousOperation (MO)/Subsystem1 ==
  Constant : Constant
  Out1 : Outport
  wires:
  Constant/1 -> Out1/1

== system LabFabSim2022a__2_9_2023_AllAttacks_/NetworkScan/InitNetScan ==
  note: On Entry: Generate 2 NetScan attack entities
  Entity Generator1 : EntityGenerator  InputPortMessageModes=m  OutputPortMessageModes=m  GenerationMethod=Event-based  Period=inf  AttributeName=data  EntityType=Structured  EntityTypeName=InitNetScan
      settings: InputPortMap=u0
  Entity Terminator2 : EntityTerminator  InputPortMessageModes=m  EntryAction=|  NumberEntitiesArrived=on
      | for i = 1:2
      |     NetScanGen();
      | end
      settings: OutputPortMap=o0
  Simulink Function2 : Subsystem  TreatAsAtomicUnit=on
  Subsystem2 : Subsystem
  Out1 : Outport
  wires:
  Subsystem2/1(Out1) -> Simulink Function2/1(In1)
  Simulink Function2/1(Out1) -> Entity Generator1/1
  Entity Terminator2/1 -> Out1/1
  Entity Generator1/1 -> Entity Terminator2/1

== system LabFabSim2022a__2_9_2023_AllAttacks_/NetworkScan/NetScan ==
  NetScan : TriggerPort  TriggerType=function-call  IsSimulinkFunction=on  FunctionName=NetScan  VariantControl=(inherit)
  Message Send : Send  OutputPortMessageModes=m
  u : ArgIn  DisableCoverage=on  ArgumentName=u
  Out1 : Outport
  wires:
  u/1 -> Message Send/1
  Message Send/1 -> Out1/1

== system LabFabSim2022a__2_9_2023_AllAttacks_/NetworkScan/Simulink Function1 ==
  In1 : Inport
  NetScanGen : TriggerPort  TriggerType=function-call  IsSimulinkFunction=on  FunctionName=NetScanGen  VariantControl=(inherit)
  Message Send : Send  OutputPortMessageModes=m
  Out1 : Outport
  wires:
  Message Send/1 -> Out1/1
  In1/1 -> Message Send/1

== system LabFabSim2022a__2_9_2023_AllAttacks_/NetworkScan/Subsystem1 ==
  Constant : Constant
  Out1 : Outport
  wires:
  Constant/1 -> Out1/1

== system LabFabSim2022a__2_9_2023_AllAttacks_/Part Ordering/Simulink Function ==
  TimeStamp() : TriggerPort  TriggerType=function-call  IsSimulinkFunction=on  FunctionName=TimeStamp  VariantControl=(inherit)
  Digital Clock : DigitalClock  SampleTime=-1
  y : ArgOut  DisableCoverage=on  ArgumentName=y
  wires:
  Digital Clock/1 -> y/1

== system LabFabSim2022a__2_9_2023_AllAttacks_/Part Ordering/Simulink Function1 ==
  In1 : Inport
  EntityGen : TriggerPort  TriggerType=function-call  IsSimulinkFunction=on  FunctionName=EntityGen  VariantControl=(inherit)
  Message Send : Send  OutputPortMessageModes=m
  Out1 : Outport
  wires:
  Message Send/1 -> Out1/1
  In1/1 -> Message Send/1

== system LabFabSim2022a__2_9_2023_AllAttacks_/Part Ordering/Simulink Function2 ==
  In1 : Inport
  OrderGen() : TriggerPort  TriggerType=function-call  IsSimulinkFunction=on  FunctionName=OrderGen  VariantControl=(inherit)
  Message Send : Send  OutputPortMessageModes=m
  Out1 : Outport
  wires:
  Message Send/1 -> Out1/1
  In1/1 -> Message Send/1

== system LabFabSim2022a__2_9_2023_AllAttacks_/Part Ordering/Simulink Function3 ==
  ReleaseEntity : TriggerPort  TriggerType=function-call  IsSimulinkFunction=on  FunctionName=ReleaseEntity  VariantControl=(inherit)
  Constant : Constant
  Message Send : Send  OutputPortMessageModes=m
  Out1 : Outport
  wires:
  Constant/1 -> Message Send/1
  Message Send/1 -> Out1/1

== system LabFabSim2022a__2_9_2023_AllAttacks_/Part Ordering/Subsystem1 ==
  Constant : Constant
  Out1 : Outport
  wires:
  Constant/1 -> Out1/1

== system LabFabSim2022a__2_9_2023_AllAttacks_/Part Ordering/Subsystem3 ==
  Constant : Constant
  Out1 : Outport
  wires:
  Constant/1 -> Out1/1

== system LabFabSim2022a__2_9_2023_AllAttacks_/SLD (Network Scan)/Simulink Function ==
  InitVGRproc2() : TriggerPort  TriggerType=function-call  IsSimulinkFunction=on  FunctionName=InitVGRproc2  VariantControl=(inherit)
  Constant : Constant
  Message Send : Send  OutputPortMessageModes=m
  Out1 : Outport
  wires:
  Constant/1 -> Message Send/1
  Message Send/1 -> Out1/1

== system LabFabSim2022a__2_9_2023_AllAttacks_/SLD (Network Scan)/Simulink Function2 ==
  NetScan_Router : TriggerPort  TriggerType=function-call  IsSimulinkFunction=on  FunctionName=NetScan_Router  VariantControl=(inherit)
  Constant : Constant  Value=2
  Constant1 : Constant
  Switch : Switch  Threshold=2  ZeroCross=off  SaturateOnIntegerOverflow=off  InputSameDT=off
  u : ArgIn  DisableCoverage=on  ArgumentName=u
  Out1 : Outport
  wires:
  u/1 -> Switch/2
  Switch/1 -> Out1/1
  Constant1/1 -> Switch/1
  Constant/1 -> Switch/3

== system LabFabSim2022a__2_9_2023_AllAttacks_/Spying/InitSpying ==
  note: On Entry: Generate 5 Spying attack entities
  Entity Generator1 : EntityGenerator  InputPortMessageModes=m  OutputPortMessageModes=m  GenerationMethod=Event-based  Period=inf  AttributeName=data  EntityType=Structured  EntityTypeName=InitSpying
      settings: InputPortMap=u0
  Entity Terminator2 : EntityTerminator  InputPortMessageModes=m  EntryAction=|  NumberEntitiesArrived=on
      | for i = 1:5
      |     SpyingGen();
      | end
      settings: OutputPortMap=o0
  Simulink Function2 : Subsystem  TreatAsAtomicUnit=on
  Subsystem2 : Subsystem
  Out1 : Outport
  wires:
  Subsystem2/1(Out1) -> Simulink Function2/1(In1)
  Simulink Function2/1(Out1) -> Entity Generator1/1
  Entity Terminator2/1 -> Out1/1
  Entity Generator1/1 -> Entity Terminator2/1

== system LabFabSim2022a__2_9_2023_AllAttacks_/Spying/Simulink Function1 ==
  In1 : Inport
  SpyingGen : TriggerPort  TriggerType=function-call  IsSimulinkFunction=on  FunctionName=SpyingGen  VariantControl=(inherit)
  Message Send : Send  OutputPortMessageModes=m
  Out1 : Outport
  wires:
  Message Send/1 -> Out1/1
  In1/1 -> Message Send/1
